simulink model "Nonlinear_system_control"  (R2021b)
settings: Solver=VariableStepAuto  StartTime=0.0  StopTime=10  RelTol=1e-3
settings Model: Creator=98744  LastModifiedBy=98744

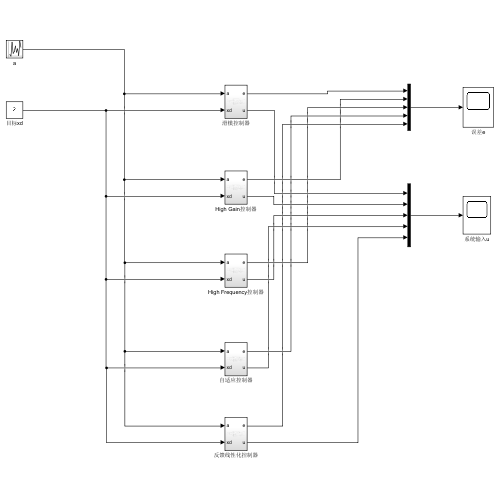
[thumbnail: Simulink's stored preview of the top-level diagram]
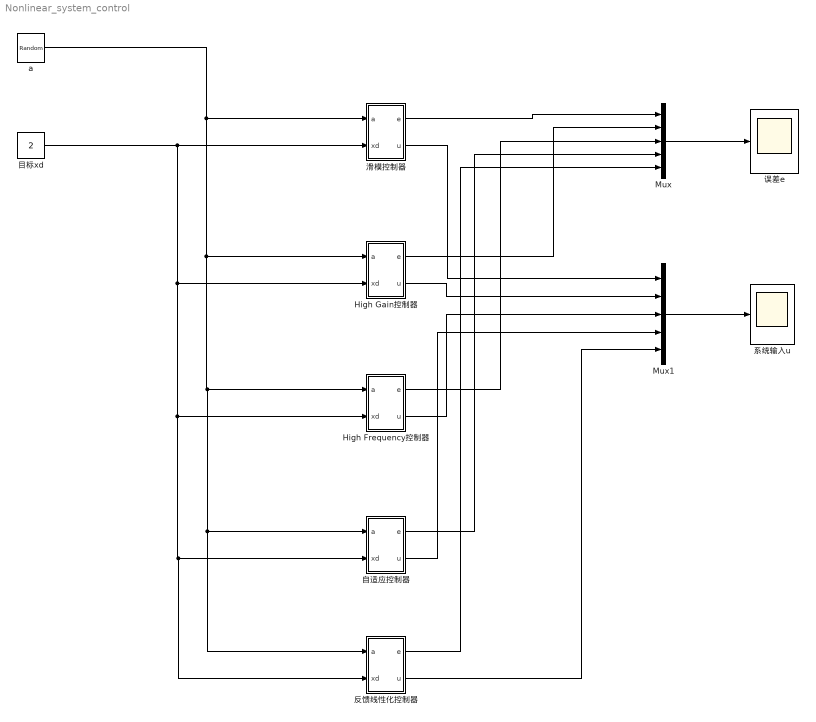
== system Nonlinear_system_control ==
  High Frequency控制器 : Subsystem
  High Gain控制器 : Subsystem
  Mux : Mux  Inputs=5
  Mux1 : Mux  Inputs=5
  a : UniformRandomNumber  SampleTime=0.1
  反馈线性化控制器 : Subsystem
  滑模控制器 : Subsystem
  目标xd : Constant  Value=2
  系统输入u : Scope
  自适应控制器 : Subsystem
  误差e : Scope
  wires:
  a/1 -> 反馈线性化控制器/1(a), 自适应控制器/1(a), High Frequency控制器/1(a), High Gain控制器/1(a), 滑模控制器/1(a)
  目标xd/1 -> 反馈线性化控制器/2(xd), 自适应控制器/2(xd), High Frequency控制器/2(xd), High Gain控制器/2(xd), 滑模控制器/2(xd)
  滑模控制器/2(u) -> Mux1/1
  High Gain控制器/2(u) -> Mux1/2
  Mux1/1 -> 系统输入u/1
  滑模控制器/1(e) -> Mux/1
  High Gain控制器/1(e) -> Mux/2
  Mux/1 -> 误差e/1
  High Frequency控制器/1(e) -> Mux/3
  High Frequency控制器/2(u) -> Mux1/3
  自适应控制器/1(e) -> Mux/4
  自适应控制器/2(u) -> Mux1/4
  反馈线性化控制器/1(e) -> Mux/5
  反馈线性化控制器/2(u) -> Mux1/5

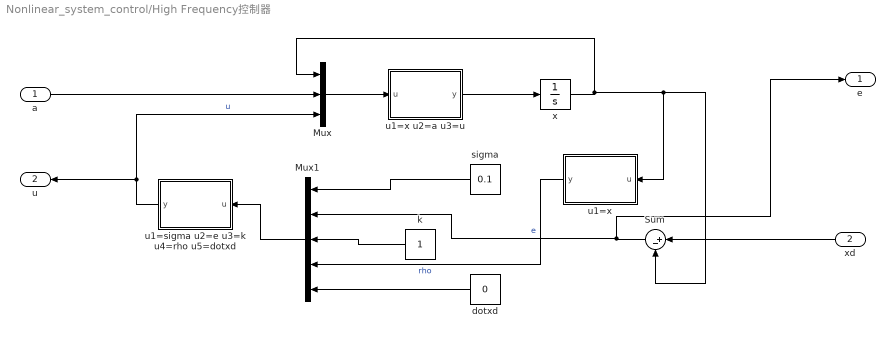
== system Nonlinear_system_control/High Frequency控制器 ==
  a : Inport
  xd : Inport  Port=2
  Mux : Mux  Inputs=[1 1 1]
  Mux1 : Mux  Inputs=5
  Sum : Sum  Inputs=|+-
  dotxd : Constant  Value=0
  k : Constant
  sigma : Constant  Value=0.1
  u1=sigma u2=e u3=k u4=rho u5=dotxd : MATLAB Function  TreatAsAtomicUnit=on
  u1=x : MATLAB Function  TreatAsAtomicUnit=on
  u1=x u2=a u3=u : MATLAB Function  TreatAsAtomicUnit=on
  x : Integrator
  e : Outport
  u : Outport  Port=2
  wires:
  sigma/1 -> Mux1/1
  xd/1 -> Sum/1
  dotxd/1 -> Mux1/5
  u1=x/1(y) -> Mux1/4  "rho"
  a/1 -> Mux/2
  Mux/1 -> u1=x u2=a u3=u/1(u)
  k/1 -> Mux1/3
  x/1 -> Mux/1, Sum/2, u1=x/1(u)
  u1=sigma u2=e u3=k u4=rho u5=dotxd/1(y) -> Mux/3, u/1  "u"
  Sum/1 -> Mux1/2, e/1  "e"
  u1=x u2=a u3=u/1(y) -> x/1
  Mux1/1 -> u1=sigma u2=e u3=k u4=rho u5=dotxd/1(u)

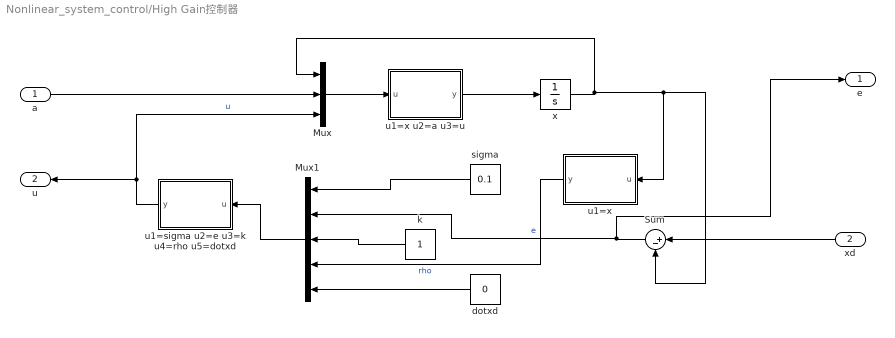
== system Nonlinear_system_control/High Gain控制器 ==
  a : Inport
  xd : Inport  Port=2
  Mux : Mux  Inputs=[1 1 1]
  Mux1 : Mux  Inputs=5
  Sum : Sum  Inputs=|+-
  dotxd : Constant  Value=0
  k : Constant
  sigma : Constant  Value=0.1
  u1=sigma u2=e u3=k u4=rho u5=dotxd : MATLAB Function  TreatAsAtomicUnit=on
  u1=x : MATLAB Function  TreatAsAtomicUnit=on
  u1=x u2=a u3=u : MATLAB Function  TreatAsAtomicUnit=on
  x : Integrator
  e : Outport
  u : Outport  Port=2
  wires:
  Mux1/1 -> u1=sigma u2=e u3=k u4=rho u5=dotxd/1(u)
  u1=x u2=a u3=u/1(y) -> x/1
  Sum/1 -> e/1, Mux1/2  "e"
  u1=sigma u2=e u3=k u4=rho u5=dotxd/1(y) -> u/1, Mux/3  "u"
  x/1 -> u1=x/1(u), Sum/2, Mux/1
  k/1 -> Mux1/3
  Mux/1 -> u1=x u2=a u3=u/1(u)
  a/1 -> Mux/2
  u1=x/1(y) -> Mux1/4  "rho"
  dotxd/1 -> Mux1/5
  xd/1 -> Sum/1
  sigma/1 -> Mux1/1

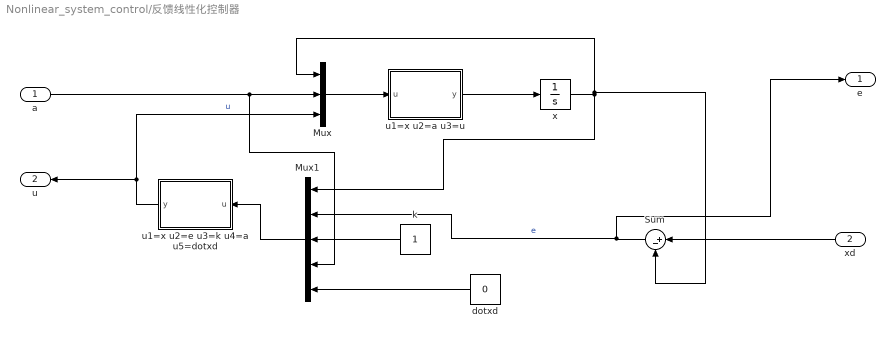
== system Nonlinear_system_control/反馈线性化控制器 ==
  a : Inport
  xd : Inport  Port=2
  Mux : Mux  Inputs=[1 1 1]
  Mux1 : Mux  Inputs=5
  Sum : Sum  Inputs=|+-
  dotxd : Constant  Value=0
  k : Constant
  u1=x u2=a u3=u : MATLAB Function  TreatAsAtomicUnit=on
  u1=x u2=e u3=k u4=a u5=dotxd : MATLAB Function  TreatAsAtomicUnit=on
  x : Integrator
  e : Outport
  u : Outport  Port=2
  wires:
  xd/1 -> Sum/1
  dotxd/1 -> Mux1/5
  a/1 -> Mux1/4, Mux/2
  Mux/1 -> u1=x u2=a u3=u/1(u)
  k/1 -> Mux1/3
  x/1 -> Mux1/1, Mux/1, Sum/2
  u1=x u2=e u3=k u4=a u5=dotxd/1(y) -> Mux/3, u/1  "u"
  Sum/1 -> Mux1/2, e/1  "e"
  u1=x u2=a u3=u/1(y) -> x/1
  Mux1/1 -> u1=x u2=e u3=k u4=a u5=dotxd/1(u)

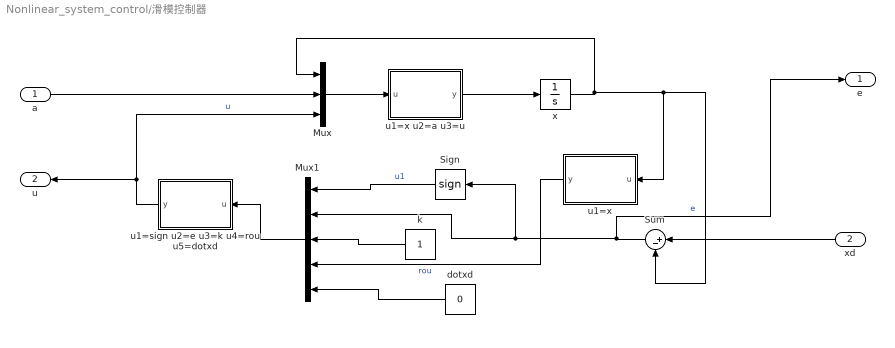
== system Nonlinear_system_control/滑模控制器 ==
  a : Inport
  xd : Inport  Port=2
  Mux : Mux  Inputs=[1 1 1]
  Mux1 : Mux  Inputs=5
  Sign : Signum  ZeroCross=off
  Sum : Sum  Inputs=|+-
  dotxd : Constant  Value=0
  k : Constant
  u1=sign u2=e u3=k u4=rou u5=dotxd : MATLAB Function  TreatAsAtomicUnit=on
  u1=x : MATLAB Function  TreatAsAtomicUnit=on
  u1=x u2=a u3=u : MATLAB Function  TreatAsAtomicUnit=on
  x : Integrator
  e : Outport
  u : Outport  Port=2
  wires:
  Mux1/1 -> u1=sign u2=e u3=k u4=rou u5=dotxd/1(u)
  u1=x u2=a u3=u/1(y) -> x/1
  Sum/1 -> e/1, Mux1/2, Sign/1  "e"
  u1=sign u2=e u3=k u4=rou u5=dotxd/1(y) -> u/1, Mux/3  "u"
  x/1 -> u1=x/1(u), Sum/2, Mux/1
  k/1 -> Mux1/3
  Sign/1 -> Mux1/1  "u1"
  Mux/1 -> u1=x u2=a u3=u/1(u)
  a/1 -> Mux/2
  u1=x/1(y) -> Mux1/4  "rou"
  dotxd/1 -> Mux1/5
  xd/1 -> Sum/1

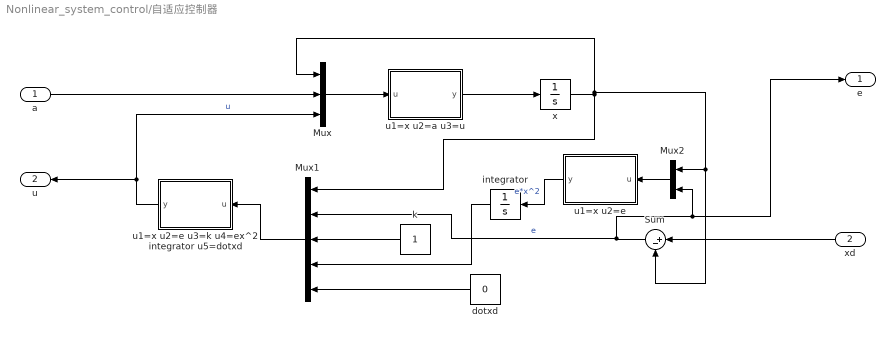
== system Nonlinear_system_control/自适应控制器 ==
  a : Inport
  xd : Inport  Port=2
  Mux : Mux  Inputs=[1 1 1]
  Mux1 : Mux  Inputs=5
  Mux2 : Mux  Inputs=2
  Sum : Sum  Inputs=|+-
  dotxd : Constant  Value=0
  integrator : Integrator
  k : Constant
  u1=x u2=a u3=u : MATLAB Function  TreatAsAtomicUnit=on
  u1=x u2=e : MATLAB Function  TreatAsAtomicUnit=on
  u1=x u2=e u3=k u4=ex^2 integrator u5=dotxd : MATLAB Function  TreatAsAtomicUnit=on
  x : Integrator
  e : Outport
  u : Outport  Port=2
  wires:
  Mux1/1 -> u1=x u2=e u3=k u4=ex^2 integrator u5=dotxd/1(u)
  u1=x u2=a u3=u/1(y) -> x/1
  Sum/1 -> Mux2/2, e/1, Mux1/2  "e"
  u1=x u2=e u3=k u4=ex^2 integrator u5=dotxd/1(y) -> u/1, Mux/3  "u"
  x/1 -> Mux2/1, Sum/2, Mux/1, Mux1/1
  k/1 -> Mux1/3
  Mux/1 -> u1=x u2=a u3=u/1(u)
  a/1 -> Mux/2
  dotxd/1 -> Mux1/5
  xd/1 -> Sum/1
  u1=x u2=e/1(y) -> integrator/1  "e*x^2"
  integrator/1 -> Mux1/4
  Mux2/1 -> u1=x u2=e/1(u)

== matlab function Nonlinear_system_control/滑模控制器/u1=x u2=a u3=u ==
  data: u input; y output
function y = fcn(u)

y = u(2)*u(1)^2+u(3);

== matlab function Nonlinear_system_control/滑模控制器/u1=x ==
  data: u input; y output
function y = fcn(u)

y = u(1)^2+0.1;

== matlab function Nonlinear_system_control/High Gain控制器/u1=sigma u2=e u3=k u4=rho u5=dotxd ==
  data: u input; y output
function y = fcn(u)

y = u(4)^2*u(2)/u(1)+u(2)*u(3)+u(5);

== matlab function Nonlinear_system_control/High Gain控制器/u1=x ==
  data: u input; y output
function y = fcn(u)

y = u(1)^2+0.1;

== matlab function Nonlinear_system_control/High Gain控制器/u1=x u2=a u3=u ==
  data: u input; y output
function y = fcn(u)

y = u(2)*u(1)^2+u(3);

== matlab function Nonlinear_system_control/High Frequency控制器/u1=sigma u2=e u3=k u4=rho u5=dotxd ==
  data: u input; y output
function y = fcn(u)

y = u(4)^2*u(2)/(u(1)+u(4)*abs(u(2)))+u(2)*u(3)+u(5);

== matlab function Nonlinear_system_control/High Frequency控制器/u1=x ==
  data: u input; y output
function y = fcn(u)

y = u(1)^2+0.1;

== matlab function Nonlinear_system_control/High Frequency控制器/u1=x u2=a u3=u ==
  data: u input; y output
function y = fcn(u)

y = u(2)*u(1)^2+u(3);

== matlab function Nonlinear_system_control/滑模控制器/u1=sign u2=e u3=k u4=rou u5=dotxd ==
  data: u input; y output
function y = fcn(u)

y = u(1)*u(4)+u(2)*u(3)+u(5);

== matlab function Nonlinear_system_control/自适应控制器/u1=x u2=e u3=k u4=ex^2 integrator u5=dotxd ==
  data: u input; y output
function y = fcn(u)

y = u(1)^2*u(4)+u(2)*u(3)+u(5);

== matlab function Nonlinear_system_control/自适应控制器/u1=x u2=e ==
  data: u input; y output
function y = fcn(u)

y = u(1)^2*u(2);

== matlab function Nonlinear_system_control/自适应控制器/u1=x u2=a u3=u ==
  data: u input; y output
function y = fcn(u)

y = u(2)*u(1)^2+u(3);

== matlab function Nonlinear_system_control/反馈线性化控制器/u1=x u2=a u3=u ==
  data: u input; y output
function y = fcn(u)

y = u(2)*u(1)^2+u(3);

== matlab function Nonlinear_system_control/反馈线性化控制器/u1=x u2=e u3=k u4=a u5=dotxd ==
  data: u input; y output
function y = fcn(u)

y = -u(1)^2*u(4)+u(2)*u(3)+u(5);
